simulink model "lab7"  (R2013b)
settings: Solver=ode3  StartTime=0.0  StopTime=15  FixedStep=0.01  RelTol=1e-3
libraries: simulink x3
settings Model: Creator=Niirn  LastModifiedBy=Niirn

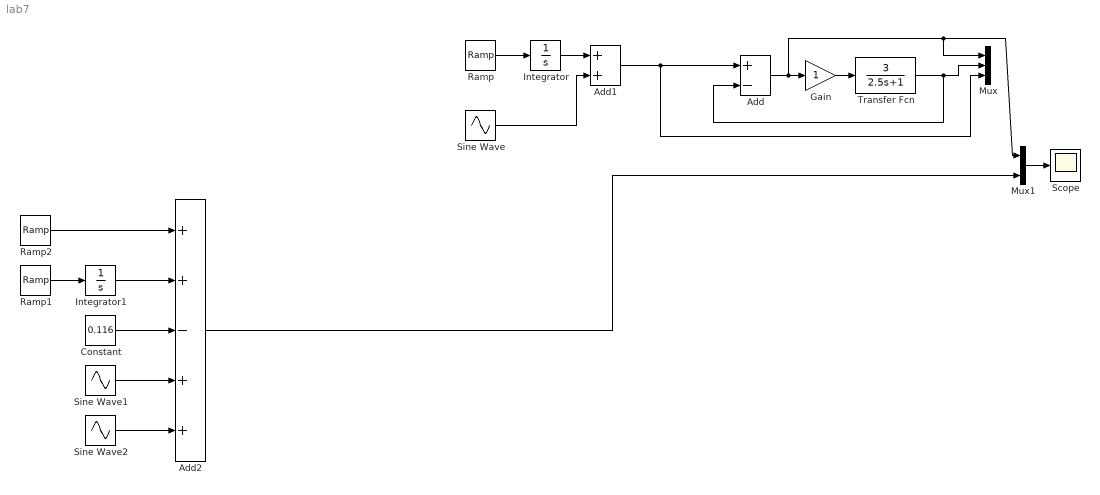
== system lab7 ==
  Add : Sum  Inputs=+-
  Add1 : Sum
  Add2 : Sum  Inputs=++-++
  Constant : Constant  Value=0.116
  Gain : Gain
  Integrator : Integrator
  Integrator1 : Integrator
  Mux : Mux  Inputs=3
  Mux1 : Mux  Inputs=2
  Ramp : simulink/Sources/Ramp  slope=0.4  start=0  X0=0
  Ramp1 : simulink/Sources/Ramp  slope=0.1  start=0  X0=0
  Ramp2 : simulink/Sources/Ramp  slope=0.188  start=0  X0=0
  Scope : Scope
      settings: ShowLegends=on  TimeRange=5  YMin=0  YMax=1
  Sine Wave : Sin  Frequency=0.5  SampleTime=0
  Sine Wave1 : Sin  Amplitude=0.3225  Frequency=0.5  SampleTime=0
  Sine Wave2 : Sin  Amplitude=0.235  Frequency=0.5  Phase=pi/2  SampleTime=0
  Transfer Fcn : TransferFcn  Numerator=[3]  Denominator=[2.5 1]
  wires:
  Transfer Fcn/1 -> Mux/2, Add/2
  Ramp/1 -> Integrator/1
  Add/1 -> Gain/1, Mux1/1, Mux/1
  Gain/1 -> Transfer Fcn/1
  Integrator/1 -> Add1/1
  Sine Wave/1 -> Add1/2
  Ramp1/1 -> Integrator1/1
  Integrator1/1 -> Add2/2
  Ramp2/1 -> Add2/1
  Add1/1 -> Mux/3, Add/1
  Constant/1 -> Add2/3
  Sine Wave1/1 -> Add2/4
  Sine Wave2/1 -> Add2/5
  Mux1/1 -> Scope/1
  Add2/1 -> Mux1/2
